simulink model "freego_jump"  (R2022b)
settings: Solver=ode15s  StartTime=0.0  StopTime=20  FixedStep=0.0001  MaxStep=0.04  MinStep=1e-10  RelTol=1e-3  EnableMultiTasking=on
model workspace (MATLAB code in the model file):
  | model = quadruped_robot();
undefined symbols (not defined in the file or in its folder): abad_InitAngle, Fpt, freego, gcontact, gcPosVel, hip_InitAngle, knee_InitAngle, quadruped_robot
libraries: simulink x5, slpidlib x2
(part 1 of 2)
settings Model: Creator=roy  LastModifiedBy=crown133
settings SolverCC: AlgebraicLoopSolver=TrustRegion
settings DataIOCC: SaveFormat=Array  SignalLoggingSaveFormat=ModelDataLogs  ReturnWorkspaceOutputs=off
settings OptimizationCC: ExpressionDepthLimit=2147483647  InitFltsAndDblsToZero=on  LifeSpan=inf
settings DebuggingCC: UnderspecifiedInitializationDetection=Classic  MergeDetectMultiDrivingBlocksExec=none  SolverPrmCheckMsg=warning  FcnCallInpInsideContextMsg=warning  UnconnectedInputMsg=warning  UnconnectedOutputMsg=warning  UnconnectedLineMsg=warning  StateNameClashWarn=warning  SFUnexpectedBacktrackingDiag=warning  SFNoUnconditionalDefaultTransitionDiag=warning  SFExecutionAtInitializationDiag=none  SFMachineParentedDataDiag=warning  ArithmeticOperatorsInVariantConditions=warning
settings HardwareCC: ProdBitPerPointer=32  ProdBitPerSizeT=32  ProdBitPerPtrDiffT=32  ProdLargestAtomicFloat=None  ProdIntDivRoundTo=Undefined  ProdEndianess=Unspecified  ProdWordSize=32  ProdHWDeviceType=32-bit Generic
settings ModelReferenceCC: EnableRefExpFcnMdlSchedulingChecks=on  PropagateSignalLabelsOutOfModel=off
settings SFSimCC: SimUseLocalCustomCode=off  CustomCodeUndefinedFunction=UseInterfaceOnly
settings RTWCC: RTWUseLocalCustomCode=off
settings CodeAppCC: StateflowObjectComments=on
settings GRTTargetCC: TargetLangStandard=C89/C90 (ANSI)  CombineOutputUpdateFcns=off  GRTInterface=on
settings ConfigComp: CovMetricSettings=dw  CovSaveCumulativeToWorkspaceVar=on  CovSaveSingleToWorkspaceVar=on  CovExternalEMLEnable=off

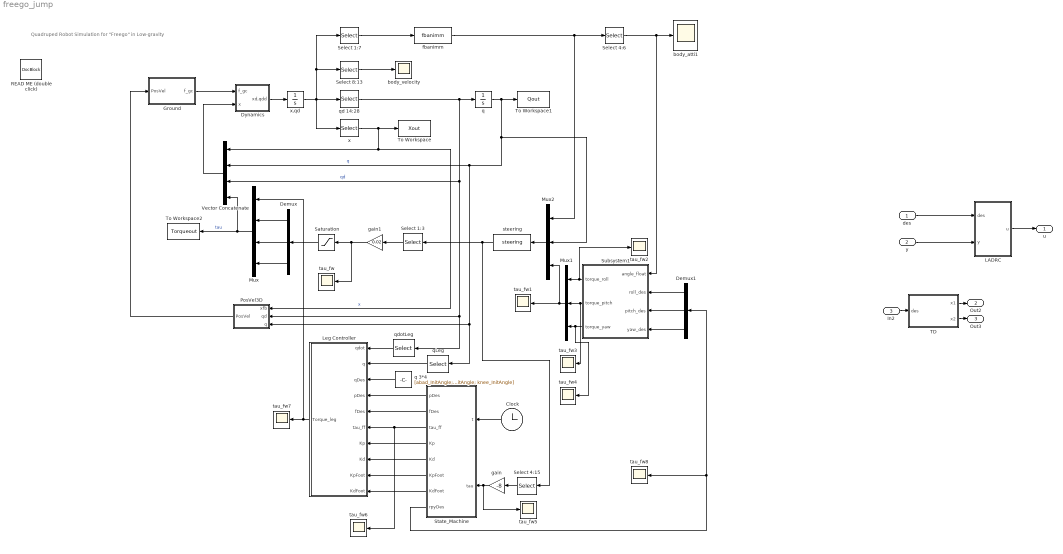
== system freego_jump ==
  note: Quadruped Robot Simulation for "Freego" in Low-gravity
  des : Inport
  y : Inport  Port=2
  In2 : Inport  Port=3
  Clock : Clock
  Demux : Demux  Outputs=3
  Demux1 : Demux  Outputs=3
  Dynamics : Subsystem
  Ground : Subsystem
  LADRC : Subsystem
  Leg Controller : Subsystem
  Mux : Mux
  Mux1 : Mux  Inputs=3
  Mux2 : Mux  Inputs=3
  PosVel3D : Subsystem
  READ ME (double click) : simulink/Model-Wide Utilities/DocBlock  DocumentType=Text
      content=|
      | This Simulink model shows how to use the ground-contact model, which
      | allows you to simulate the effect of physical contact between a rigid-body
      | system and a compliant ground plane.
      |
      | showmotion(quadruped_robot(), tout, fbanim(Xout, Qout))
      |
      | fbanim() 专为showmotion() 设计
  Saturation : Saturate  UpperLimit=1  LowerLimit=-1
  Select 1:3 : Selector  InputPortWidth=15  IndexOptions=Index vector (dialog)  Indices=[1:3]  OutputSizes=1
  Select 1:7 : Selector  InputPortWidth=13+15  IndexOptions=Index vector (dialog)  Indices=[1:7]  OutputSizes=1
  Select 4:15 : Selector  InputPortWidth=15  IndexOptions=Index vector (dialog)  Indices=[4:15]  OutputSizes=1
  Select 4:6 : Selector  InputPortWidth=6  IndexOptions=Index vector (dialog)  Indices=[4:6]  OutputSizes=1
  Select 8:13 : Selector  InputPortWidth=13+15  IndexOptions=Index vector (dialog)  Indices=[8 9 10 11 12 13]  OutputSizes=1
  State_Machine : Subsystem
  Subsystem1 : Subsystem
  TD : Subsystem
  To Workspace : ToWorkspace  VariableName=Xout  SampleTime=-1
  To Workspace1 : ToWorkspace  VariableName=Qout  SampleTime=-1
  To Workspace2 : ToWorkspace  VariableName=Torqueout  SampleTime=-1
  Vector Concatenate : Concatenate  NumInputs=4
  body_atti1 : Scope
  body_velocity : Scope
  fbanimm : MATLABFcn  MATLABFcn=fbanimm  OutputDimensions=6
  gain : Gain  Gain=-8
  gain1 : Gain  Gain=0.02
  q : Integrator  InitialCondition=[freego.q_init]'
  q 3*4 : Constant  Value=[abad_InitAngle; hip_InitAngle; knee_InitAngle]
  qLeg : Selector  InputPortWidth=15  IndexOptions=Index vector (dialog)  Indices=[1:12]  OutputSizes=1
  qd 14:28 : Selector  InputPortWidth=13+15  IndexOptions=Index vector (dialog)  Indices=[14:13+15]  OutputSizes=1
  qdotLeg : Selector  InputPortWidth=15  IndexOptions=Index vector (dialog)  Indices=[1:12]  OutputSizes=1
  steering : MATLABFcn  MATLABFcn=steering  OutputDimensions=15  Output1D=off
  tau_fw{,1..8} (9 alike) : Scope
  x : Selector  InputPortWidth=13+15  IndexOptions=Index vector (dialog)  Indices=[1:13]  OutputSizes=1
  x,qd : Integrator  InitialCondition=[freego.QuatBody, freego.COMLocation, zeros(1,6), zeros(1,15)]'
  u : Outport
  Out2 : Outport  Port=2
  Out3 : Outport  Port=3
  wires:
  PosVel3D/1(PosVel) -> Ground/1(PosVel)
  Dynamics/1(xd,qdd) -> x,qd/1
  Select 8:13/1 -> body_velocity/1
  qd 14:28/1 -> q/1, qdotLeg/1, PosVel3D/2(qd), Vector Concatenate/3  "qd"
  q/1 -> To Workspace1/1, Mux2/2, Vector Concatenate/2, qLeg/1, PosVel3D/3(q)  "q"
  x/1 -> To Workspace/1, Vector Concatenate/1, PosVel3D/1(xfb)  "x"
  Vector Concatenate/1 -> Dynamics/2(x)
  Ground/1(f_gc) -> Dynamics/1(f_gc)
  Mux/1 -> Vector Concatenate/4, To Workspace2/1  "tau"
  des/1 -> LADRC/1(des)
  y/1 -> LADRC/2(y)
  LADRC/1(u) -> u/1
  In2/1 -> TD/1(des)
  TD/2(x2) -> Out3/1
  TD/1(x1) -> Out2/1
  Demux/1 -> Mux/2
  q 3*4/1 -> Leg Controller/3(qDes)
  Leg Controller/1(Torque_leg) -> Mux/1, tau_fw7/1
  qLeg/1 -> Leg Controller/2(q)
  qdotLeg/1 -> Leg Controller/1(qdot)
  Select 1:7/1 -> fbanimm/1
  fbanimm/1 -> Select 4:6/1, Mux2/1
  Select 4:6/1 -> body_atti1/1, Subsystem1/1(angle_float)
  Demux1/2 -> Subsystem1/3(pitch_des)
  Subsystem1/1(torque_roll) -> Mux1/1, tau_fw2/1
  Subsystem1/2(torque_pitch) -> Mux1/2, tau_fw3/1
  Subsystem1/3(torque_yaw) -> Mux1/3, tau_fw4/1
  Mux2/1 -> steering/1
  Mux1/1 -> tau_fw1/1, Mux2/3
  steering/1 -> Select 4:15/1, Select 1:3/1
  Select 1:3/1 -> gain1/1
  gain1/1 -> tau_fw/1, Saturation/1
  Select 4:15/1 -> gain/1
  Demux1/1 -> Subsystem1/2(roll_des)
  Demux1/3 -> Subsystem1/4(yaw_des)
  Saturation/1 -> Demux/1
  Clock/1 -> State_Machine/1(t)
  gain/1 -> tau_fw5/1, State_Machine/2(tau)
  State_Machine/7(KdFoot) -> Leg Controller/10(KdFoot)
  State_Machine/6(KpFoot) -> Leg Controller/9(KpFoot)
  State_Machine/5(Kd) -> Leg Controller/8(Kd)
  State_Machine/4(Kp) -> Leg Controller/7(Kp)
  State_Machine/3(tau_ff) -> tau_fw6/1, Leg Controller/6(tau_ff)
  State_Machine/2(fDes) -> Leg Controller/5(fDes)
  State_Machine/1(pDes) -> Leg Controller/4(pDes)
  State_Machine/8(rpyDes) -> tau_fw8/1, Demux1/1
  Demux/3 -> Mux/4
  Demux/2 -> Mux/3
  x,qd/1 -> x/1, qd 14:28/1, Select 1:7/1, Select 8:13/1

== system freego_jump/Dynamics ==
  f_gc : Inport
  x : Inport  Port=2
  Quadruped_robot Dynamics : MATLABFcn  MATLABFcn=gcFD( quadruped_robot, @FDfb, u )  OutputDimensions=[13+15 1]  OutputSignalType=real  Output1D=off
  Reshape : Reshape  OutputDimensionality=Column vector (2-D)
  Vector Concatenate : Concatenate
  xd,qdd : Outport
  wires:
  Vector Concatenate/1 -> Quadruped_robot Dynamics/1
  Quadruped_robot Dynamics/1 -> xd,qdd/1
  f_gc/1 -> Reshape/1
  x/1 -> Vector Concatenate/1
  Reshape/1 -> Vector Concatenate/2

== system freego_jump/Ground ==
  PosVel : Inport
  3D Ground Contact : Subsystem  mask(3D Nonlinear Ground Contact with Friction){K=1e6, D=2000, mu=0.35, np=16}
      mask prompts: K "Stiffness (K)"; D "Damping (D)"; mu "Coefficient of Friction (mu)"; np "Number of Contact Points"
      mask help:
      | Given two 3xnp arrays containing contact-point positions and
      | velocities, calculate the 3xnp array of ground-reaction forces
      | acting on those points. Also calculate 1xnp boolean vectors
      | in_ctact (true if normal force >0) and sticking (true if inside
      | or on boundary of friction cone).  Zero-crossing detection is
      | enabled at both make/break contact and stick/slip transitions.
  READ ME : simulink/Model-Wide Utilities/DocBlock  DocumentType=Text
      content=|
      | This subsystem implements the Simulink ground-contact model in 3D.  The
      | input is a 6x(npt) matrix such that column i contains the 3D position (top
      | 3 elements) and linear velocity (bottom 3 elements) of ground-contact
      | point number i (i.e., the i^th point defined in the "gc" field of the
      | system model data structure).  The output is a 6x(npt) matrix such that
      | column i is the spatial force acting on point number i.  All quantities
      | are expressed in base (body 0) coordinates.
      |
      | The first thing that happens is that the input matrix is split into
      | separate position and velocity matrices.  Both are then sent to the "3D
      | Ground Contact" subsystem, which calculates the force acting on each
      | point.  The "force" output is a 3x(npt) matrix of linear forces, which is
      | converted to a matrix of spatial forces by the final block in the
      | subsystem.  The other two outputs are 1x(npt) arrays of Boolean variables
      | such that in_ctact(i) is true if point i is in contact with the ground
      | (meaning that it is experiencing a nonzero force) and sticking(i) is true
      | if point i is sticking (due to friction) to the ground.
      |
      | The subsystem "3D Ground Contact" is a masked subsystem.  If you
      | double-click on this block then you will get a dialog window displaying
      | the following parameters: Stiffness (K), Damping (D), coefficient of
      | friction (mu), and Number of Contact Points.  The first three must be
      | strictly-positive scalars, and the fourth must equal the number of points
      | defined in the "gc" field of the system model data structure.  The current
      | settings of K, D and mu correspond to a soft, very slippery plastic
      | surface.  Increasing K will make it harder, and increasing the ratio K/D
      | will make it bouncier, but be aware that both increase the stiffness of
      | the differential equations that Simulink is solving, meaning that Simulink
      | will be forced to take smaller steps.  A typical value of mu for a safe
      | (non-slip) floor is 0.5.
      |
      | To see how this subsystem is implemented, you will have to look under the
      | mask.  You can do that by right-clicking on the block and selecting the
      | menu option "Look Under Mask".  There, you will find that this block is
      | based on the function gcontact, and you will also find a bit more
      | documentation.
  Terminator : Terminator
  Terminator1 : Terminator
  convert 3D to spatial forces : Subsystem
  select pos : Selector  NumberOfDimensions=2  InputPortWidth=3  IndexOptions=Index vector (dialog),Select all  Indices=[1 2 3],1  OutputSizes=1,1
  select vel : Selector  NumberOfDimensions=2  InputPortWidth=3  IndexOptions=Index vector (dialog),Select all  Indices=[4 5 6],1  OutputSizes=1,1
  f_gc : Outport
  wires:
  PosVel/1 -> select pos/1, select vel/1
  select pos/1 -> convert 3D to spatial forces/1(pos), 3D Ground Contact/1(pos)
  convert 3D to spatial forces/1(force6D) -> f_gc/1
  select vel/1 -> 3D Ground Contact/2(vel)
  3D Ground Contact/1(force) -> convert 3D to spatial forces/2(force3D)
  3D Ground Contact/2(in_ctact) -> Terminator/1
  3D Ground Contact/3(sticking) -> Terminator1/1

== system freego_jump/LADRC ==
  des : Inport
  y : Inport  Port=2
  1/b0 : Gain
  LESO3 : Subsystem
  PID Controller : slpidlib/PID Controller  Controller=PID  Form=Parallel  TimeDomain=Continuous-time  UseExternalTs=off  SampleTime=-1  IntegratorMethod=Forward Euler  FilterMethod=Forward Euler  ControllerParametersSource=internal  P=10  I=0.01  UseKiTs=off  D=1  N=100  UseFilter=on  TunerSelectOption=Transfer Function Based (PID Tuner App)  InitialConditionSource=internal  InitialConditionForIntegrator=0  InitialConditionForFilter=0  DifferentiatorICPrevScaledInput=0  ExternalReset=none  TrackingMode=off  Kt=1  LimitOutput=off  SatLimitsSource=internal  UpperSaturationLimit=inf  LowerSaturationLimit=-inf  LinearizeAsGain=on  AntiWindupMode=none  Kb=1  LimitIntegrator=off  UpperIntegratorSaturationLimit=inf  LowerIntegratorSaturationLimit=-inf  POutMin=[]  POutMax=[]  IOutMin=[]  IOutMax=[]  DOutMin=[]  DOutMax=[]  NOutMin=[]  NOutMax=[]  SumOutMin=[]  SumOutMax=[]  SaturationOutMin=[]  SaturationOutMax=[]  PParamMin=[]  PParamMax=[]  IParamMin=[]  IParamMax=[]  DParamMin=[]  DParamMax=[]  NParamMin=[]  NParamMax=[]  KbParamMin=[]  KbParamMax=[]  KtParamMin=[]  KtParamMax=[]  KbOutMin=[]  KbOutMax=[]  KtOutMin=[]  KtOutMax=[]  IntegratorOutMin=[]  IntegratorOutMax=[]  FilterOutMin=[]  FilterOutMax=[]  SumI1OutMin=[]  SumI1OutMax=[]  SumI2OutMin=[]  SumI2OutMax=[]  SumI3OutMin=[]  SumI3OutMax=[]  SumI4OutMin=[]  SumI4OutMax=[]  SumDOutMin=[]  SumDOutMax=[]  DifferentiatorOutMin=[]  DifferentiatorOutMax=[]  FilterDiffOutCoefMin=[]  FilterDiffOutCoefMax=[]  ReciprocalOutMin=[]  ReciprocalOutMax=[]  SumDenOutMin=[]  SumDenOutMax=[]  SumNumOutMin=[]  SumNumOutMax=[]  DivideOutMin=[]  DivideOutMax=[]  UdiffTsProdOutMin=[]  UdiffTsProdOutMax=[]  NTsProdOutMin=[]  NTsProdOutMax=[]  UintegralTsProdOutMin=[]  UintegralTsProdOutMax=[]  UngainTsProdOutMin=[]  UngainTsProdOutMax=[]  ClampingZeroOutDataTypeStr=Inherit: Inherit via back propagation  ClampingZeroOutMin=[]  ClampingZeroOutMax=[]  FilterDenConstantOutDataTypeStr=Inherit: Inherit via back propagation  FilterDenConstantOutMin=[]  FilterDenConstantOutMax=[]  PCopyOutDataTypeStr=Inherit: Inherit via back propagation  PCopyOutMin=[]  PCopyOutMax=[]  NCopyOutDataTypeStr=Inherit: Inherit via back propagation  NCopyOutMin=[]  NCopyOutMax=[]  IntegratorContinuousStateAttributes=''  IntegratorStateMustResolveToSignalObject=off  IntegratorRTWStateStorageClass=Auto  FilterContinuousStateAttributes=''  FilterStateMustResolveToSignalObject=off  FilterRTWStateStorageClass=Auto  ParallelPVariant=InternalParameters  IdealPVariant=Disabled  IVariant=InternalParameters  DVariant=InternalParameters  IntegratorVariant=Continuous  SatVariant=Disabled  AWVariant=Passthrough  PCopyVariant=Disabled  TRVariant=Disabled  FdbkBlocksVariant=Forward  IdealPFdbkVariant=Disabled  SatFdbkVariant=Disabled  DerivativeFilterVariant=ContFilter  NVariant=InternalParameters  NCopyVariant=Disabled  FilterICVariant=InternalICsFilter  IntegratorICVariant=InternalICs  ExternalResetVariant=Disabled  TRSumVariant=Passthrough  SumFdbkVariant=Disabled  SumVariant=Sum_PID  TsampFilterVariant=InternalTs  TsampNgainVariant=Passthrough  TsampIntegralVariant=Passthrough  ExternalSaturationOutDataTypeStr=Inherit: Same as second input
  PID Controller1 : slpidlib/PID Controller  Controller=PID  Form=Parallel  TimeDomain=Continuous-time  UseExternalTs=off  SampleTime=-1  IntegratorMethod=Forward Euler  FilterMethod=Forward Euler  ControllerParametersSource=internal  P=10  I=0.01  UseKiTs=off  D=1  N=100  UseFilter=on  TunerSelectOption=Transfer Function Based (PID Tuner App)  InitialConditionSource=internal  InitialConditionForIntegrator=0  InitialConditionForFilter=0  DifferentiatorICPrevScaledInput=0  ExternalReset=none  TrackingMode=off  Kt=1  LimitOutput=off  SatLimitsSource=internal  UpperSaturationLimit=inf  LowerSaturationLimit=-inf  LinearizeAsGain=on  AntiWindupMode=none  Kb=1  LimitIntegrator=off  UpperIntegratorSaturationLimit=inf  LowerIntegratorSaturationLimit=-inf  POutMin=[]  POutMax=[]  IOutMin=[]  IOutMax=[]  DOutMin=[]  DOutMax=[]  NOutMin=[]  NOutMax=[]  SumOutMin=[]  SumOutMax=[]  SaturationOutMin=[]  SaturationOutMax=[]  PParamMin=[]  PParamMax=[]  IParamMin=[]  IParamMax=[]  DParamMin=[]  DParamMax=[]  NParamMin=[]  NParamMax=[]  KbParamMin=[]  KbParamMax=[]  KtParamMin=[]  KtParamMax=[]  KbOutMin=[]  KbOutMax=[]  KtOutMin=[]  KtOutMax=[]  IntegratorOutMin=[]  IntegratorOutMax=[]  FilterOutMin=[]  FilterOutMax=[]  SumI1OutMin=[]  SumI1OutMax=[]  SumI2OutMin=[]  SumI2OutMax=[]  SumI3OutMin=[]  SumI3OutMax=[]  SumI4OutMin=[]  SumI4OutMax=[]  SumDOutMin=[]  SumDOutMax=[]  DifferentiatorOutMin=[]  DifferentiatorOutMax=[]  FilterDiffOutCoefMin=[]  FilterDiffOutCoefMax=[]  ReciprocalOutMin=[]  ReciprocalOutMax=[]  SumDenOutMin=[]  SumDenOutMax=[]  SumNumOutMin=[]  SumNumOutMax=[]  DivideOutMin=[]  DivideOutMax=[]  UdiffTsProdOutMin=[]  UdiffTsProdOutMax=[]  NTsProdOutMin=[]  NTsProdOutMax=[]  UintegralTsProdOutMin=[]  UintegralTsProdOutMax=[]  UngainTsProdOutMin=[]  UngainTsProdOutMax=[]  ClampingZeroOutDataTypeStr=Inherit: Inherit via back propagation  ClampingZeroOutMin=[]  ClampingZeroOutMax=[]  FilterDenConstantOutDataTypeStr=Inherit: Inherit via back propagation  FilterDenConstantOutMin=[]  FilterDenConstantOutMax=[]  PCopyOutDataTypeStr=Inherit: Inherit via back propagation  PCopyOutMin=[]  PCopyOutMax=[]  NCopyOutDataTypeStr=Inherit: Inherit via back propagation  NCopyOutMin=[]  NCopyOutMax=[]  IntegratorContinuousStateAttributes=''  IntegratorStateMustResolveToSignalObject=off  IntegratorRTWStateStorageClass=Auto  FilterContinuousStateAttributes=''  FilterStateMustResolveToSignalObject=off  FilterRTWStateStorageClass=Auto  ParallelPVariant=InternalParameters  IdealPVariant=Disabled  IVariant=InternalParameters  DVariant=InternalParameters  IntegratorVariant=Continuous  SatVariant=Disabled  AWVariant=Passthrough  PCopyVariant=Disabled  TRVariant=Disabled  FdbkBlocksVariant=Forward  IdealPFdbkVariant=Disabled  SatFdbkVariant=Disabled  DerivativeFilterVariant=ContFilter  NVariant=InternalParameters  NCopyVariant=Disabled  FilterICVariant=InternalICsFilter  IntegratorICVariant=InternalICs  ExternalResetVariant=Disabled  TRSumVariant=Passthrough  SumFdbkVariant=Disabled  SumVariant=Sum_PID  TsampFilterVariant=InternalTs  TsampNgainVariant=Passthrough  TsampIntegralVariant=Passthrough  ExternalSaturationOutDataTypeStr=Inherit: Same as second input
  Sum1 : Sum  Inputs=|+-
  Sum2 : Sum  Inputs=|+-
  Sum3 : Sum  Inputs=+|+
  Sum4 : Sum  Inputs=|+-
  "TD3 " : Subsystem
  b0 : Gain
  u : Outport
  wires:
  des/1 -> "TD3 "/1(des)
  Sum3/1 -> Sum4/1
  1/b0/1 -> Sum4/2
  PID Controller1/1 -> Sum3/2
  y/1 -> LESO3/1(y)
  Sum2/1 -> PID Controller1/1
  LESO3/3(z3) -> 1/b0/1
  PID Controller/1 -> Sum3/1
  "TD3 "/2(x2) -> Sum2/1
  LESO3/2(z2) -> Sum2/2
  "TD3 "/1(x1) -> Sum1/1
  Sum1/1 -> PID Controller/1
  b0/1 -> LESO3/2(b0u)
  LESO3/1(z1) -> Sum1/2
  Sum4/1 -> u/1, b0/1

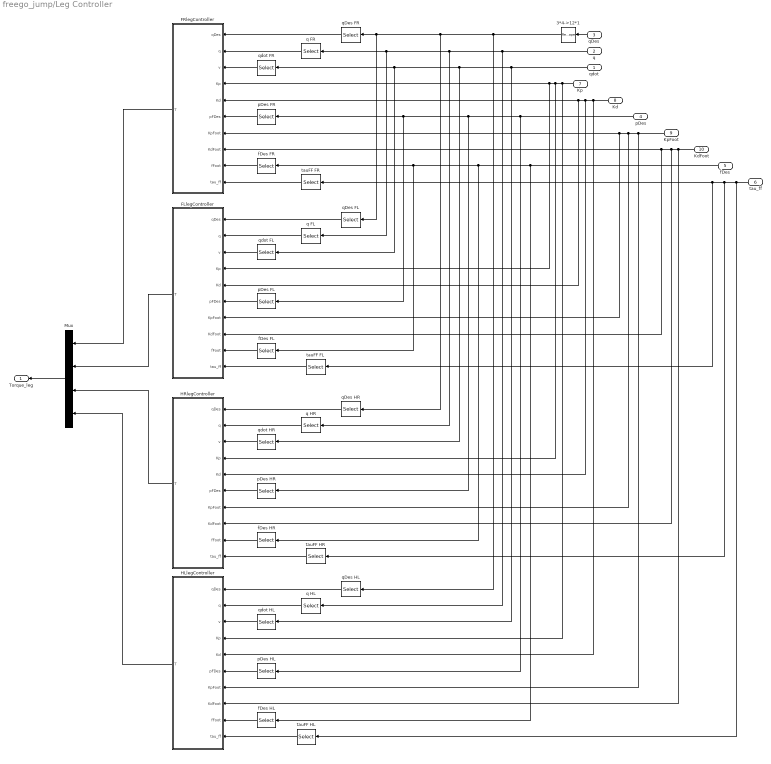
== system freego_jump/Leg Controller ==
  qdot : Inport
  q : Inport  Port=2
  qDes : Inport  Port=3
  pDes : Inport  Port=4
  fDes : Inport  Port=5
  tau_ff : Inport  Port=6
  Kp : Inport  Port=7
  Kd : Inport  Port=8
  KpFoot : Inport  Port=9
  KdFoot : Inport  Port=10
  3*4->12*1 : Reshape  OutputDimensionality=Column vector (2-D)
  FLlegController : Subsystem
  FRlegController : Subsystem
  HLlegController : Subsystem
  HRlegController : Subsystem
  Mux : Mux
  fDes FL : Selector  InputPortWidth=12  IndexOptions=Index vector (dialog)  Indices=[4:6]  OutputSizes=1
  fDes FR : Selector  InputPortWidth=12  IndexOptions=Index vector (dialog)  Indices=[1:3]  OutputSizes=1
  fDes HL : Selector  InputPortWidth=12  IndexOptions=Index vector (dialog)  Indices=[10:12]  OutputSizes=1
  fDes HR : Selector  InputPortWidth=12  IndexOptions=Index vector (dialog)  Indices=[7:9]  OutputSizes=1
  pDes FL : Selector  InputPortWidth=12  IndexOptions=Index vector (dialog)  Indices=[4:6]  OutputSizes=1
  pDes FR : Selector  InputPortWidth=12  IndexOptions=Index vector (dialog)  Indices=[1:3]  OutputSizes=1
  pDes HL : Selector  InputPortWidth=12  IndexOptions=Index vector (dialog)  Indices=[10:12]  OutputSizes=1
  pDes HR : Selector  InputPortWidth=12  IndexOptions=Index vector (dialog)  Indices=[7:9]  OutputSizes=1
  q FL : Selector  InputPortWidth=12  IndexOptions=Index vector (dialog)  Indices=[4:6]  OutputSizes=1
  q FR : Selector  InputPortWidth=12  IndexOptions=Index vector (dialog)  Indices=[1:3]  OutputSizes=1
  q HL : Selector  InputPortWidth=12  IndexOptions=Index vector (dialog)  Indices=[10:12]  OutputSizes=1
  q HR : Selector  InputPortWidth=12  IndexOptions=Index vector (dialog)  Indices=[7:9]  OutputSizes=1
  qDes FL : Selector  InputPortWidth=12  IndexOptions=Index vector (dialog)  Indices=[4:6]  OutputSizes=1
  qDes FR : Selector  InputPortWidth=12  IndexOptions=Index vector (dialog)  Indices=[1:3]  OutputSizes=1
  qDes HL : Selector  InputPortWidth=12  IndexOptions=Index vector (dialog)  Indices=[10:12]  OutputSizes=1
  qDes HR : Selector  InputPortWidth=12  IndexOptions=Index vector (dialog)  Indices=[7:9]  OutputSizes=1
  qdot FL : Selector  InputPortWidth=12  IndexOptions=Index vector (dialog)  Indices=[4:6]  OutputSizes=1
  qdot FR : Selector  InputPortWidth=12  IndexOptions=Index vector (dialog)  Indices=[1:3]  OutputSizes=1
  qdot HL : Selector  InputPortWidth=12  IndexOptions=Index vector (dialog)  Indices=[10:12]  OutputSizes=1
  qdot HR : Selector  InputPortWidth=12  IndexOptions=Index vector (dialog)  Indices=[7:9]  OutputSizes=1
  tauFF FL : Selector  InputPortWidth=12  IndexOptions=Index vector (dialog)  Indices=[4:6]  OutputSizes=1
  tauFF FR : Selector  InputPortWidth=12  IndexOptions=Index vector (dialog)  Indices=[1:3]  OutputSizes=1
  tauFF HL : Selector  InputPortWidth=12  IndexOptions=Index vector (dialog)  Indices=[10:12]  OutputSizes=1
  tauFF HR : Selector  InputPortWidth=12  IndexOptions=Index vector (dialog)  Indices=[7:9]  OutputSizes=1
  Torque_leg : Outport
  wires:
  q FR/1 -> FRlegController/2(q)
  qDes/1 -> 3*4->12*1/1
  qdot/1 -> qdot FL/1, qdot FR/1, qdot HR/1, qdot HL/1
  qdot FR/1 -> FRlegController/3(v)
  q FL/1 -> FLlegController/2(q)
  Kd/1 -> HLlegController/5(Kd), HRlegController/5(Kd), FRlegController/5(Kd), FLlegController/5(Kd)
  KpFoot/1 -> FRlegController/7(KpFoot), FLlegController/7(KpFoot), HRlegController/7(KpFoot), HLlegController/7(KpFoot)
  qDes FL/1 -> FLlegController/1(qDes)
  pDes FL/1 -> FLlegController/6(pFDes)
  q/1 -> q FL/1, q FR/1, q HR/1, q HL/1
  qdot FL/1 -> FLlegController/3(v)
  qDes FR/1 -> FRlegController/1(qDes)
  pDes FR/1 -> FRlegController/6(pFDes)
  3*4->12*1/1 -> qDes FL/1, qDes FR/1, qDes HR/1, qDes HL/1
  pDes/1 -> pDes FL/1, pDes FR/1, pDes HR/1, pDes HL/1
  q HR/1 -> HRlegController/2(q)
  qDes HR/1 -> HRlegController/1(qDes)
  pDes HR/1 -> HRlegController/6(pFDes)
  qdot HR/1 -> HRlegController/3(v)
  q HL/1 -> HLlegController/2(q)
  Kp/1 -> HLlegController/4(Kp), HRlegController/4(Kp), FLlegController/4(Kp), FRlegController/4(Kp)
  KdFoot/1 -> FRlegController/8(KdFoot), FLlegController/8(KdFoot), HRlegController/8(KdFoot), HLlegController/8(KdFoot)
  fDes/1 -> fDes HL/1, fDes HR/1, fDes FL/1, fDes FR/1
  qDes HL/1 -> HLlegController/1(qDes)
  pDes HL/1 -> HLlegController/6(pFDes)
  qdot HL/1 -> HLlegController/3(v)
  Mux/1 -> Torque_leg/1
  FRlegController/1(T) -> Mux/1
  FLlegController/1(T) -> Mux/2
  HRlegController/1(T) -> Mux/3
  HLlegController/1(T) -> Mux/4
  fDes FR/1 -> FRlegController/9(fFoot)
  fDes FL/1 -> FLlegController/9(fFoot)
  fDes HR/1 -> HRlegController/9(fFoot)
  fDes HL/1 -> HLlegController/9(fFoot)
  tauFF FL/1 -> FLlegController/10(tau_ff)
  tauFF HR/1 -> HRlegController/10(tau_ff)
  tauFF HL/1 -> HLlegController/10(tau_ff)
  tauFF FR/1 -> FRlegController/10(tau_ff)
  tau_ff/1 -> tauFF HL/1, tauFF HR/1, tauFF FL/1, tauFF FR/1

== system freego_jump/PosVel3D ==
  note: The constant supplies the
      | argument for rollingdisc
  xfb : Inport
  qd : Inport  Port=2
  q : Inport  Port=3
  Vector Concatenate1 : Concatenate  NumInputs=3
  gcPosVel : MATLABFcn  MATLABFcn=gcPosVel( quadruped_robot(), u(1:13), u(14:28), u(29:43))  OutputDimensions=[6 16]  OutputSignalType=real  Output1D=off
  PosVel : Outport
  wires:
  gcPosVel/1 -> PosVel/1
  Vector Concatenate1/1 -> gcPosVel/1
  q/1 -> Vector Concatenate1/2
  xfb/1 -> Vector Concatenate1/1
  qd/1 -> Vector Concatenate1/3

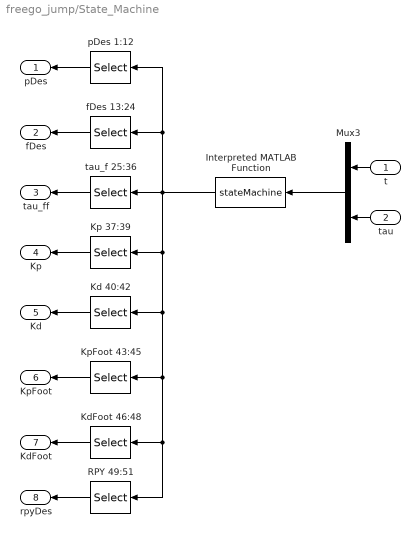
== system freego_jump/State_Machine ==
  t : Inport
  tau : Inport  Port=2
  Interpreted MATLAB Function : MATLABFcn  MATLABFcn=stateMachine  OutputDimensions=51
  Kd 40:42 : Selector  InputPortWidth=51  IndexOptions=Index vector (dialog)  Indices=[40:42]  OutputSizes=1
  KdFoot 46:48 : Selector  InputPortWidth=51  IndexOptions=Index vector (dialog)  Indices=[46:48]  OutputSizes=1
  Kp 37:39 : Selector  InputPortWidth=51  IndexOptions=Index vector (dialog)  Indices=[37:39]  OutputSizes=1
  KpFoot 43:45 : Selector  InputPortWidth=51  IndexOptions=Index vector (dialog)  Indices=[43:45]  OutputSizes=1
  Mux3 : Mux  Inputs=2
  RPY 49:51 : Selector  InputPortWidth=51  IndexOptions=Index vector (dialog)  Indices=[49:51]  OutputSizes=1
  fDes 13:24 : Selector  InputPortWidth=51  IndexOptions=Index vector (dialog)  Indices=[13:24]  OutputSizes=1
  pDes 1:12 : Selector  InputPortWidth=51  IndexOptions=Index vector (dialog)  Indices=[1:12]  OutputSizes=1
  tau_f 25:36 : Selector  InputPortWidth=51  IndexOptions=Index vector (dialog)  Indices=[25:36]  OutputSizes=1
  pDes : Outport
  fDes : Outport  Port=2
  tau_ff : Outport  Port=3
  Kp : Outport  Port=4
  Kd : Outport  Port=5
  KpFoot : Outport  Port=6
  KdFoot : Outport  Port=7
  rpyDes : Outport  Port=8
  wires:
  pDes 1:12/1 -> pDes/1
  fDes 13:24/1 -> fDes/1
  tau/1 -> Mux3/2
  t/1 -> Mux3/1
  tau_f 25:36/1 -> tau_ff/1
  Interpreted MATLAB Function/1 -> pDes 1:12/1, fDes 13:24/1, tau_f 25:36/1, Kp 37:39/1, Kd 40:42/1, KpFoot 43:45/1, RPY 49:51/1, KdFoot 46:48/1
  Mux3/1 -> Interpreted MATLAB Function/1
  Kp 37:39/1 -> Kp/1
  Kd 40:42/1 -> Kd/1
  KpFoot 43:45/1 -> KpFoot/1
  KdFoot 46:48/1 -> KdFoot/1
  RPY 49:51/1 -> rpyDes/1

== system freego_jump/Subsystem1 ==
  angle_float : Inport
  roll_des : Inport  Port=2
  pitch_des : Inport  Port=3
  yaw_des : Inport  Port=4
  Demux : Demux  Outputs=3
  LADRC_Pitch : Subsystem
  LADRC_Roll : Subsystem
  LADRC_Yaw : Subsystem
  p : Gain  Gain=-1
  p1 : Gain  Gain=-1
  p2 : Gain  Gain=-1
  torque_roll : Outport
  torque_pitch : Outport  Port=2
  torque_yaw : Outport  Port=3
  wires:
  LADRC_Yaw/1(u) -> p2/1
  yaw_des/1 -> LADRC_Yaw/1(des)
  pitch_des/1 -> LADRC_Pitch/1(des)
  LADRC_Pitch/1(u) -> p1/1
  angle_float/1 -> Demux/1
  p/1 -> torque_roll/1
  roll_des/1 -> LADRC_Roll/1(des)
  LADRC_Roll/1(u) -> p/1
  Demux/2 -> LADRC_Pitch/2(y)
  Demux/1 -> LADRC_Roll/2(y)
  Demux/3 -> LADRC_Yaw/2(y)
  p1/1 -> torque_pitch/1
  p2/1 -> torque_yaw/1

== system freego_jump/TD ==
  des : Inport
  MATLAB Function1 : MATLAB Function  TreatAsAtomicUnit=on
  Product : Product
  Product1 : Product
  Sum : Sum  Inputs=+-|
  h : Constant
  r : Constant  Value=10000000000000000000000000
  sx1 : Integrator
  sx2 : Integrator
  x1 : Outport
  x2 : Outport  Port=2
  wires:
  sx2/1 -> MATLAB Function1/2(x2), x2/1, Product1/1
  h/1 -> MATLAB Function1/4(h), Product/2, Product1/2  "h"
  Product/1 -> sx2/1
  MATLAB Function1/1(fh) -> Product/1
  sx1/1 -> Sum/1, x1/1
  r/1 -> MATLAB Function1/3(r)
  Product1/1 -> sx1/1
  Sum/1 -> MATLAB Function1/1(x1)
  des/1 -> Sum/2

== system freego_jump/Ground/3D Ground Contact ==
  pos : Inport
  vel : Inport  Port=2
  Compare To Constant : simulink/Logic and Bit Operations/Compare To Constant  relop=<=  const=1  OutDataTypeStr=boolean
  Compare To Zero : simulink/Logic and Bit Operations/Compare To Zero  relop=>  OutDataTypeStr=boolean
  K,D,mu : Constant  Value=[ [K; D; mu] zeros(3,np-1) ]  VectorParams1D=off
  READ ME : simulink/Model-Wide Utilities/DocBlock  DocumentType=Text
      content=|
      | The constant block supplies the parameters K, D and mu to the function
      | gcontact.  This is necessary because K, D and mu are defined in the
      | workspace of this particular masked subsystem, but the executable
      | expression in the "MATLAB Function" block does not have access to this
      | workspace, so the symbols K, D and mu cannot appear directly in the
      | executable expression.
      |
      | The ">0" block and the "<=1" block both have zero-crossing enabled.  The
      | former detects transitions between contact and non-contact, whereas the
      | latter detects transitions between sticking (due to friction) and
      | slipping.  A point can be sticking only if it is also in contact.  A
      | zero-crossing event occurs whenever any one point makes a transition.
      |
      | The state variable, u, is a 2x(np) matrix containing the horizontal
      | component of the local ground deformation for each point.  This quantity
      | is used to calculate the tangential (i.e., frictional) component of the
      | ground reaction force.
      |
      | When a point loses contact, its associated state variable, u(:,i), decays
      | to zero with a time constant of D/K.  If this ratio is small then the
      | corresponding differential equation is fast, and it is necessary to use
      | small integration time steps.  For example, if K=1e6 and D=2000 then
      | D/K=0.002 and u(:,i) decays in proportion to exp(-500t).  Increasing K
      | makes the surface stiffer, and decreasing D/K makes it bouncier, but the
      | latter also makes the post-contact recovery faster.  The degree of
      | bounciness depends on the mass of the impacting body: a heavier body will
      | bounce more.
      |
      | To adapt this subsystem to work in 2D, the only things that change are the
      | row dimensions of various matrices.  You will have to alter the row
      | selections in the executable expression in the "MATLAB Function" block,
      | and also the dimensions of its output matrix, and you will have to change
      | the row selections in the various "select" blocks.
      |
      | For more information, see "The Simulink Ground Contact Model" in the
      | spatial_v2 documentation directory.
  Vector Concatenate : Concatenate  NumInputs=4  Mode=Multidimensional array
  gcontact : MATLABFcn  MATLABFcn=gcontact( u(1,1), u(2,1), u(3,1), u(4:6,:), u(7:9,:), u(10:11,:) )  OutputDimensions=[6 np]  OutputSignalType=real  Output1D=off
  select fcone : Selector  NumberOfDimensions=2  InputPortWidth=3  IndexOptions=Index vector (dialog),Select all  Indices=[6],1  OutputSizes=1,1
  select force : Selector  NumberOfDimensions=2  InputPortWidth=3  IndexOptions=Index vector (dialog),Select all  Indices=[1 2 3],1  OutputSizes=1,1
  select fz : Selector  NumberOfDimensions=2  InputPortWidth=3  IndexOptions=Index vector (dialog),Select all  Indices=[3],1  OutputSizes=1,1
  select ud : Selector  NumberOfDimensions=2  InputPortWidth=3  IndexOptions=Index vector (dialog),Select all  Indices=[4 5],1  OutputSizes=1,1
  u : Integrator
  force : Outport
  in_ctact : Outport  Port=2
  sticking : Outport  Port=3
  wires:
  Vector Concatenate/1 -> gcontact/1
  select ud/1 -> u/1
  gcontact/1 -> select fz/1, select ud/1, select fcone/1, select force/1
  select force/1 -> force/1
  select fz/1 -> Compare To Zero/1
  Compare To Zero/1 -> in_ctact/1
  select fcone/1 -> Compare To Constant/1
  Compare To Constant/1 -> sticking/1
  u/1 -> Vector Concatenate/4
  vel/1 -> Vector Concatenate/3
  pos/1 -> Vector Concatenate/2
  K,D,mu/1 -> Vector Concatenate/1

== system freego_jump/Ground/convert 3D to spatial forces ==
  note: calculate a 6*npt matrix of spatial force vectors (one per column)
      | from a 3*npt matrix of position vectors specifying the points
      | through which the forces act, and a 3*npt matrix of force vectors
  pos : Inport
  force3D : Inport  Port=2
  Fpt : MATLABFcn  MATLABFcn=Fpt( u(4:6,:), u(1:3,:) )  OutputSignalType=real  Output1D=off
  Matrix Concatenate : Concatenate  Mode=Multidimensional array
  force6D : Outport
  wires:
  force3D/1 -> Matrix Concatenate/2
  pos/1 -> Matrix Concatenate/1
  Matrix Concatenate/1 -> Fpt/1
  Fpt/1 -> force6D/1

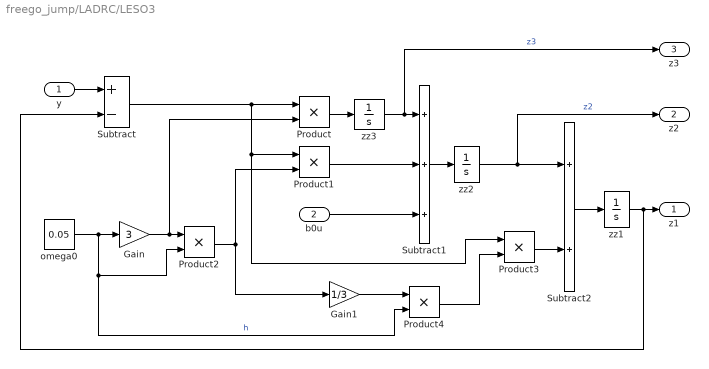
== system freego_jump/LADRC/LESO3 ==
  y : Inport
  b0u : Inport  Port=2
  Gain : Gain  Gain=3
  Gain1 : Gain  Gain=1/3
  Product{,1..4} (5 alike) : Product
  Subtract : Sum  Inputs=+-
  Subtract1 : Sum  Inputs=+++
  Subtract2 : Sum
  omega0 : Constant  Value=0.05
  zz1 : Integrator
  zz2 : Integrator
  zz3 : Integrator
  z1 : Outport
  z2 : Outport  Port=2
  z3 : Outport  Port=3
  wires:
  y/1 -> Subtract/1
  Subtract/1 -> Product/1, Product3/1, Product1/1
  omega0/1 -> Gain/1, Product4/2, Product2/2  "h"
  Gain/1 -> Product/2, Product2/1
  Product/1 -> zz3/1
  zz3/1 -> z3/1, Subtract1/1  "z3"
  b0u/1 -> Subtract1/3
  Product1/1 -> Subtract1/2
  Product2/1 -> Gain1/1, Product1/2
  Subtract1/1 -> zz2/1
  zz2/1 -> Subtract2/1, z2/1  "z2"
  zz1/1 -> Subtract/2, z1/1
  Product3/1 -> Subtract2/2
  Product4/1 -> Product3/2
  Subtract2/1 -> zz1/1
  Gain1/1 -> Product4/1

== system freego_jump/LADRC/TD3  ==
  des : Inport
  Gain : Gain  Gain=-1
  MATLAB Function1 : MATLAB Function  TreatAsAtomicUnit=on
  Product : Product
  d : Constant  Value=0.05
  r : Constant  Value=300
  sx1 : Integrator
  sx2 : Integrator
  x1 : Outport
  x2 : Outport  Port=2
  wires:
  d/1 -> MATLAB Function1/5(d)  "h"
  Product/1 -> sx2/1
  MATLAB Function1/1(f) -> Product/1
  sx1/1 -> MATLAB Function1/1(x1), x1/1
  r/1 -> Gain/1, MATLAB Function1/4(r)
  sx2/1 -> MATLAB Function1/2(x2), sx1/1, x2/1
  des/1 -> MATLAB Function1/3(u)
  Gain/1 -> Product/2

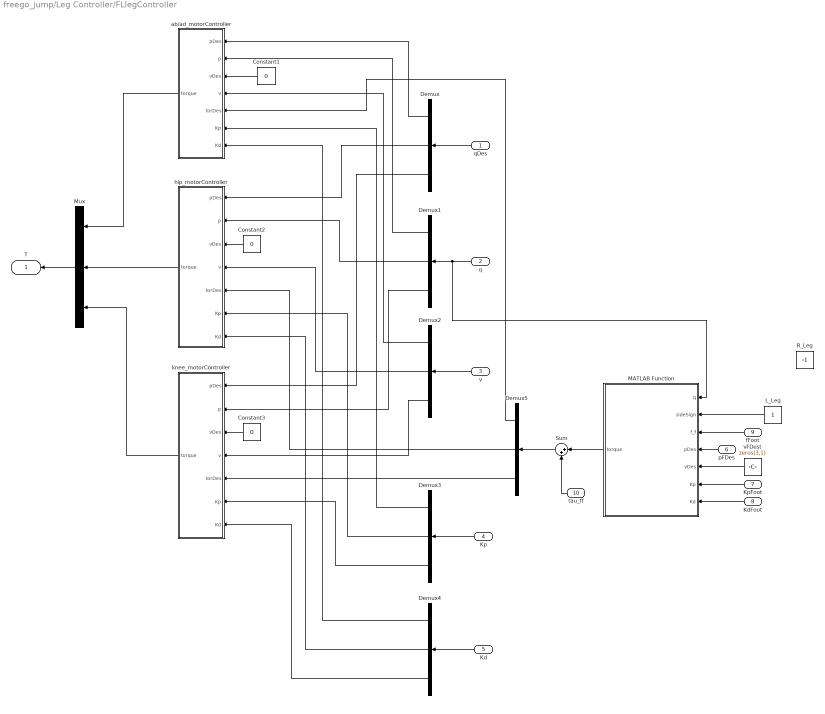
== system freego_jump/Leg Controller/FLlegController ==
  qDes : Inport
  q : Inport  Port=2
  v : Inport  Port=3
  Kp : Inport  Port=4
  Kd : Inport  Port=5
  pFDes : Inport  Port=6
  KpFoot : Inport  Port=7
  KdFoot : Inport  Port=8
  fFoot : Inport  Port=9
  tau_ff : Inport  Port=10
  Constant1 : Constant  Value=0
  Constant2 : Constant  Value=0
  Constant3 : Constant  Value=0
  Demux{,1..5} (6 alike) : Demux  Outputs=3
  L_Leg : Constant
  MATLAB Function : MATLAB Function  TreatAsAtomicUnit=on
  Mux : Mux  Inputs=3
  R_Leg : Constant  Value=-1
  Sum : Sum  Inputs=|++
  ab/ad_motorController : Subsystem
  hip_motorController : Subsystem
  knee_motorController : Subsystem
  vFDest : Constant  Value=zeros(3,1)
  T : Outport
  wires:
  Demux/1 -> ab/ad_motorController/1(pDes)
  Demux1/1 -> ab/ad_motorController/2(p)
  Demux2/1 -> ab/ad_motorController/4(v)
  Demux3/1 -> ab/ad_motorController/6(Kp)
  Demux5/1 -> ab/ad_motorController/5(torDes)
  Constant1/1 -> ab/ad_motorController/3(vDes)
  Demux4/1 -> ab/ad_motorController/7(Kd)
  ab/ad_motorController/1(torque) -> Mux/1
  Constant2/1 -> hip_motorController/3(vDes)
  Demux2/2 -> hip_motorController/4(v)
  Demux/2 -> hip_motorController/1(pDes)
  Demux1/3 -> knee_motorController/2(p)
  Demux5/2 -> hip_motorController/5(torDes)
  Demux3/2 -> hip_motorController/6(Kp)
  Demux5/3 -> knee_motorController/5(torDes)
  Demux/3 -> knee_motorController/1(pDes)
  Constant3/1 -> knee_motorController/3(vDes)
  Demux4/2 -> hip_motorController/7(Kd)
  hip_motorController/1(torque) -> Mux/2
  Demux3/3 -> knee_motorController/6(Kp)
  Demux1/2 -> hip_motorController/2(p)
  knee_motorController/1(torque) -> Mux/3
  Demux4/3 -> knee_motorController/7(Kd)
  qDes/1 -> Demux/1
  q/1 -> MATLAB Function/1(q), Demux1/1
  v/1 -> Demux2/1
  Demux2/3 -> knee_motorController/4(v)
  Kp/1 -> Demux3/1
  Kd/1 -> Demux4/1
  Mux/1 -> T/1
  fFoot/1 -> MATLAB Function/3(f_f)
  KdFoot/1 -> MATLAB Function/7(Kd)
  KpFoot/1 -> MATLAB Function/6(Kp)
  vFDest/1 -> MATLAB Function/5(vDes)
  pFDes/1 -> MATLAB Function/4(pDes)
  L_Leg/1 -> MATLAB Function/2(sideSign)
  tau_ff/1 -> Sum/2
  MATLAB Function/1(torque) -> Sum/1
  Sum/1 -> Demux5/1

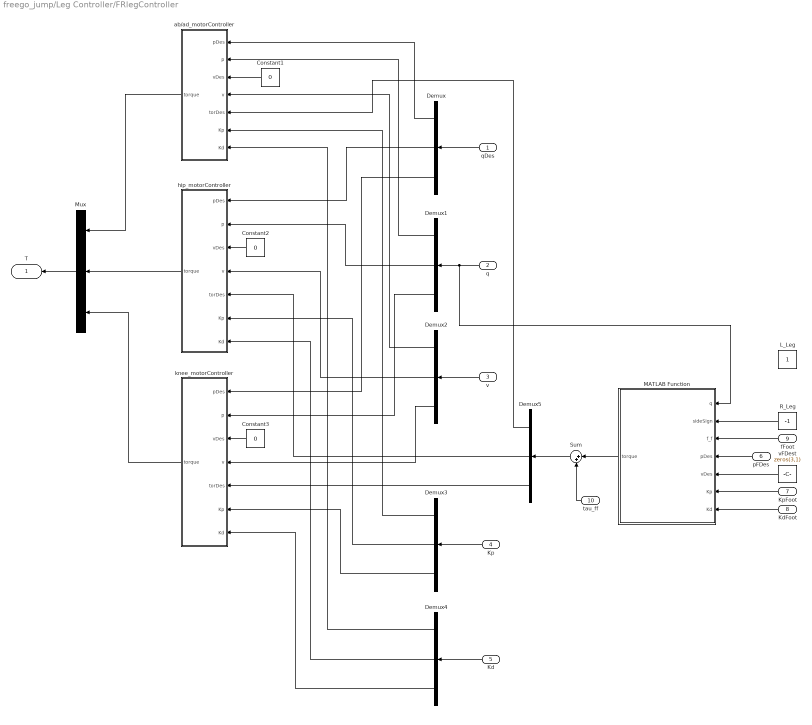
== system freego_jump/Leg Controller/FRlegController ==
  qDes : Inport
  q : Inport  Port=2
  v : Inport  Port=3
  Kp : Inport  Port=4
  Kd : Inport  Port=5
  pFDes : Inport  Port=6
  KpFoot : Inport  Port=7
  KdFoot : Inport  Port=8
  fFoot : Inport  Port=9
  tau_ff : Inport  Port=10
  Constant1 : Constant  Value=0
  Constant2 : Constant  Value=0
  Constant3 : Constant  Value=0
  Demux{,1..5} (6 alike) : Demux  Outputs=3
  L_Leg : Constant
  MATLAB Function : MATLAB Function  TreatAsAtomicUnit=on
  Mux : Mux  Inputs=3
  R_Leg : Constant  Value=-1
  Sum : Sum  Inputs=|++
  ab/ad_motorController : Subsystem
  hip_motorController : Subsystem
  knee_motorController : Subsystem
  vFDest : Constant  Value=zeros(3,1)
  T : Outport
  wires:
  Demux/1 -> ab/ad_motorController/1(pDes)
  Demux1/1 -> ab/ad_motorController/2(p)
  Demux2/1 -> ab/ad_motorController/4(v)
  Demux3/1 -> ab/ad_motorController/6(Kp)
  Demux5/1 -> ab/ad_motorController/5(torDes)
  Constant1/1 -> ab/ad_motorController/3(vDes)
  Demux4/1 -> ab/ad_motorController/7(Kd)
  ab/ad_motorController/1(torque) -> Mux/1
  Constant2/1 -> hip_motorController/3(vDes)
  Demux2/2 -> hip_motorController/4(v)
  Demux/2 -> hip_motorController/1(pDes)
  Demux1/3 -> knee_motorController/2(p)
  Demux5/2 -> hip_motorController/5(torDes)
  Demux3/2 -> hip_motorController/6(Kp)
  Demux5/3 -> knee_motorController/5(torDes)
  Demux/3 -> knee_motorController/1(pDes)
  Constant3/1 -> knee_motorController/3(vDes)
  Demux4/2 -> hip_motorController/7(Kd)
  hip_motorController/1(torque) -> Mux/2
  Demux3/3 -> knee_motorController/6(Kp)
  Demux1/2 -> hip_motorController/2(p)
  knee_motorController/1(torque) -> Mux/3
  Demux4/3 -> knee_motorController/7(Kd)
  qDes/1 -> Demux/1
  q/1 -> MATLAB Function/1(q), Demux1/1
  v/1 -> Demux2/1
  Demux2/3 -> knee_motorController/4(v)
  Kp/1 -> Demux3/1
  Kd/1 -> Demux4/1
  Mux/1 -> T/1
  fFoot/1 -> MATLAB Function/3(f_f)
  KdFoot/1 -> MATLAB Function/7(Kd)
  KpFoot/1 -> MATLAB Function/6(Kp)
  vFDest/1 -> MATLAB Function/5(vDes)
  pFDes/1 -> MATLAB Function/4(pDes)
  MATLAB Function/1(torque) -> Sum/1
  R_Leg/1 -> MATLAB Function/2(sideSign)
  tau_ff/1 -> Sum/2
  Sum/1 -> Demux5/1

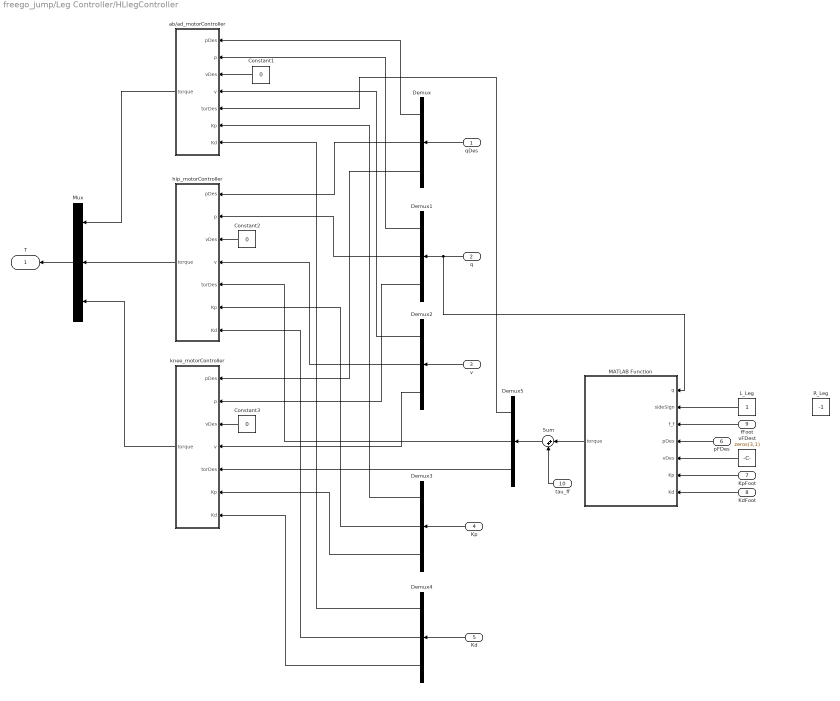
== system freego_jump/Leg Controller/HLlegController ==
  qDes : Inport
  q : Inport  Port=2
  v : Inport  Port=3
  Kp : Inport  Port=4
  Kd : Inport  Port=5
  pFDes : Inport  Port=6
  KpFoot : Inport  Port=7
  KdFoot : Inport  Port=8
  fFoot : Inport  Port=9
  tau_ff : Inport  Port=10
  Constant1 : Constant  Value=0
  Constant2 : Constant  Value=0
  Constant3 : Constant  Value=0
  Demux{,1..5} (6 alike) : Demux  Outputs=3
  L_Leg : Constant
  MATLAB Function : MATLAB Function  TreatAsAtomicUnit=on
  Mux : Mux  Inputs=3
  R_Leg : Constant  Value=-1
  Sum : Sum  Inputs=|++
  ab/ad_motorController : Subsystem
  hip_motorController : Subsystem
  knee_motorController : Subsystem
  vFDest : Constant  Value=zeros(3,1)
  T : Outport
  wires:
  Demux/1 -> ab/ad_motorController/1(pDes)
  Demux1/1 -> ab/ad_motorController/2(p)
  Demux2/1 -> ab/ad_motorController/4(v)
  Demux3/1 -> ab/ad_motorController/6(Kp)
  Demux5/1 -> ab/ad_motorController/5(torDes)
  Constant1/1 -> ab/ad_motorController/3(vDes)
  Demux4/1 -> ab/ad_motorController/7(Kd)
  ab/ad_motorController/1(torque) -> Mux/1
  Constant2/1 -> hip_motorController/3(vDes)
  Demux2/2 -> hip_motorController/4(v)
  Demux/2 -> hip_motorController/1(pDes)
  Demux1/3 -> knee_motorController/2(p)
  Demux5/2 -> hip_motorController/5(torDes)
  Demux3/2 -> hip_motorController/6(Kp)
  Demux5/3 -> knee_motorController/5(torDes)
  Demux/3 -> knee_motorController/1(pDes)
  Constant3/1 -> knee_motorController/3(vDes)
  Demux4/2 -> hip_motorController/7(Kd)
  hip_motorController/1(torque) -> Mux/2
  Demux3/3 -> knee_motorController/6(Kp)
  Demux1/2 -> hip_motorController/2(p)
  knee_motorController/1(torque) -> Mux/3
  Demux4/3 -> knee_motorController/7(Kd)
  qDes/1 -> Demux/1
  q/1 -> MATLAB Function/1(q), Demux1/1
  v/1 -> Demux2/1
  Demux2/3 -> knee_motorController/4(v)
  Kp/1 -> Demux3/1
  Kd/1 -> Demux4/1
  Mux/1 -> T/1
  fFoot/1 -> MATLAB Function/3(f_f)
  KdFoot/1 -> MATLAB Function/7(Kd)
  KpFoot/1 -> MATLAB Function/6(Kp)
  vFDest/1 -> MATLAB Function/5(vDes)
  pFDes/1 -> MATLAB Function/4(pDes)
  L_Leg/1 -> MATLAB Function/2(sideSign)
  tau_ff/1 -> Sum/2
  MATLAB Function/1(torque) -> Sum/1
  Sum/1 -> Demux5/1

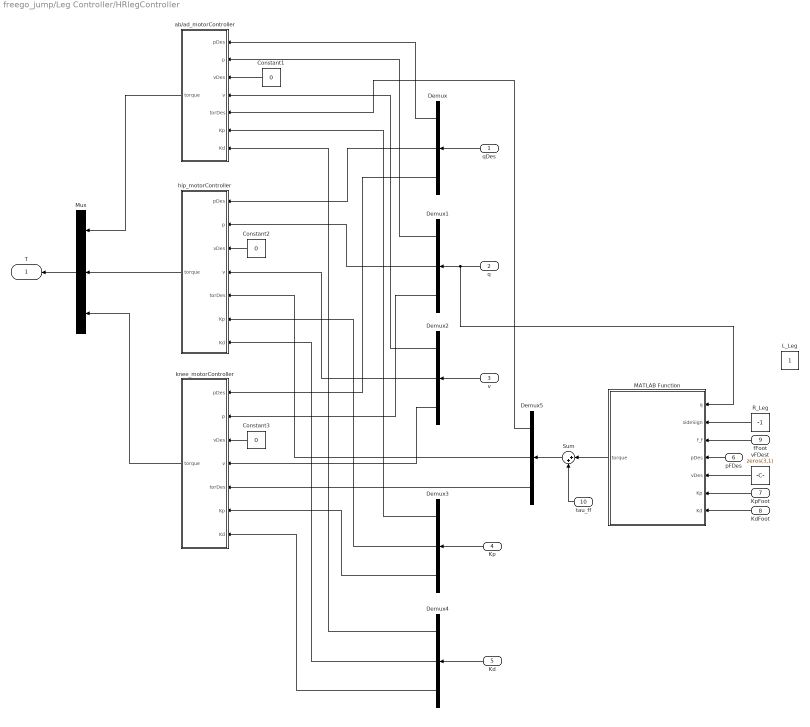
== system freego_jump/Leg Controller/HRlegController ==
  qDes : Inport
  q : Inport  Port=2
  v : Inport  Port=3
  Kp : Inport  Port=4
  Kd : Inport  Port=5
  pFDes : Inport  Port=6
  KpFoot : Inport  Port=7
  KdFoot : Inport  Port=8
  fFoot : Inport  Port=9
  tau_ff : Inport  Port=10
  Constant1 : Constant  Value=0
  Constant2 : Constant  Value=0
  Constant3 : Constant  Value=0
  Demux{,1..5} (6 alike) : Demux  Outputs=3
  L_Leg : Constant
  MATLAB Function : MATLAB Function  TreatAsAtomicUnit=on
  Mux : Mux  Inputs=3
  R_Leg : Constant  Value=-1
  Sum : Sum  Inputs=|++
  ab/ad_motorController : Subsystem
  hip_motorController : Subsystem
  knee_motorController : Subsystem
  vFDest : Constant  Value=zeros(3,1)
  T : Outport
  wires:
  Demux/1 -> ab/ad_motorController/1(pDes)
  Demux1/1 -> ab/ad_motorController/2(p)
  Demux2/1 -> ab/ad_motorController/4(v)
  Demux3/1 -> ab/ad_motorController/6(Kp)
  Demux5/1 -> ab/ad_motorController/5(torDes)
  Constant1/1 -> ab/ad_motorController/3(vDes)
  Demux4/1 -> ab/ad_motorController/7(Kd)
  ab/ad_motorController/1(torque) -> Mux/1
  Constant2/1 -> hip_motorController/3(vDes)
  Demux2/2 -> hip_motorController/4(v)
  Demux/2 -> hip_motorController/1(pDes)
  Demux1/3 -> knee_motorController/2(p)
  Demux5/2 -> hip_motorController/5(torDes)
  Demux3/2 -> hip_motorController/6(Kp)
  Demux5/3 -> knee_motorController/5(torDes)
  Demux/3 -> knee_motorController/1(pDes)
  Constant3/1 -> knee_motorController/3(vDes)
  Demux4/2 -> hip_motorController/7(Kd)
  hip_motorController/1(torque) -> Mux/2
  Demux3/3 -> knee_motorController/6(Kp)
  Demux1/2 -> hip_motorController/2(p)
  knee_motorController/1(torque) -> Mux/3
  Demux4/3 -> knee_motorController/7(Kd)
  qDes/1 -> Demux/1
  q/1 -> MATLAB Function/1(q), Demux1/1
  v/1 -> Demux2/1
  Demux2/3 -> knee_motorController/4(v)
  Kp/1 -> Demux3/1
  Kd/1 -> Demux4/1
  Mux/1 -> T/1
  fFoot/1 -> MATLAB Function/3(f_f)
  KdFoot/1 -> MATLAB Function/7(Kd)
  KpFoot/1 -> MATLAB Function/6(Kp)
  vFDest/1 -> MATLAB Function/5(vDes)
  pFDes/1 -> MATLAB Function/4(pDes)
  R_Leg/1 -> MATLAB Function/2(sideSign)
  tau_ff/1 -> Sum/2
  MATLAB Function/1(torque) -> Sum/1
  Sum/1 -> Demux5/1

== system freego_jump/Subsystem1/LADRC_Pitch ==
  des : Inport
  y : Inport  Port=2
  1/b0 : Gain  Gain=0.5
  Constant2 : Constant  Value=0
  LESO3 : Subsystem
  Sum1 : Sum  Inputs=|+-
  Sum2 : Sum  Inputs=|+-
  Sum3 : Sum  Inputs=+|+
  Sum4 : Sum  Inputs=|+-
  Zero-Pole : ZeroPole  Zeros=[0]  Poles=[-100]  Gain=[100]
  b0 : Gain  Gain=4
  body_atti{,1..3} (4 alike) : Scope  NumInputPorts=2
  d : Gain  Gain=6
  p : Gain  Gain=5
  u : Outport
  wires:
  Sum3/1 -> Sum4/1
  1/b0/1 -> body_atti2/2
  d/1 -> Sum3/2
  y/1 -> Zero-Pole/1, body_atti/2, LESO3/1(y)
  Sum2/1 -> d/1
  LESO3/3(z3) -> 1/b0/1
  p/1 -> Sum3/1
  LESO3/2(z2) -> body_atti2/1
  Sum1/1 -> p/1
  b0/1 -> LESO3/2(b0u)
  LESO3/1(z1) -> body_atti/1, Sum1/2
  Sum4/1 -> body_atti3/2, u/1, b0/1
  des/1 -> Sum1/1, body_atti1/1
  Constant2/1 -> Sum2/1, body_atti1/2
  Zero-Pole/1 -> Sum2/2

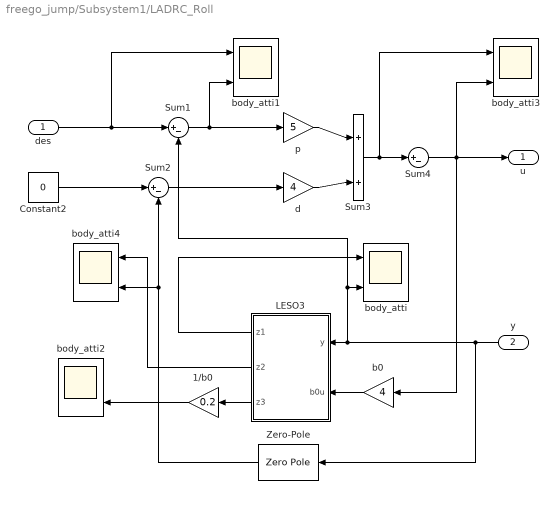
== system freego_jump/Subsystem1/LADRC_Roll ==
  des : Inport
  y : Inport  Port=2
  1/b0 : Gain  Gain=0.2
  Constant2 : Constant  Value=0
  LESO3 : Subsystem
  Sum1 : Sum  Inputs=|+-
  Sum2 : Sum  Inputs=|+-
  Sum3 : Sum  Inputs=+|+
  Sum4 : Sum  Inputs=|+-
  Zero-Pole : ZeroPole  Zeros=[0]  Poles=[-100]  Gain=[100]
  b0 : Gain  Gain=4
  body_atti{,1..4} (5 alike) : Scope  NumInputPorts=2
  d : Gain  Gain=4
  p : Gain  Gain=5
  u : Outport
  wires:
  Sum3/1 -> body_atti3/1, Sum4/1
  1/b0/1 -> body_atti2/2
  d/1 -> Sum3/2
  y/1 -> Zero-Pole/1, Sum1/2, body_atti/2, LESO3/1(y)
  Sum2/1 -> d/1
  LESO3/3(z3) -> 1/b0/1
  p/1 -> Sum3/1
  LESO3/2(z2) -> body_atti4/1
  Sum1/1 -> body_atti1/2, p/1
  b0/1 -> LESO3/2(b0u)
  LESO3/1(z1) -> body_atti/1
  Sum4/1 -> body_atti3/2, u/1, b0/1
  des/1 -> body_atti1/1, Sum1/1
  Constant2/1 -> Sum2/1
  Zero-Pole/1 -> body_atti4/2, Sum2/2

== system freego_jump/Subsystem1/LADRC_Yaw ==
  des : Inport
  y : Inport  Port=2
  1/b0 : Gain  Gain=0.5
  Constant2 : Constant  Value=0
  LESO3 : Subsystem
  Sum1 : Sum  Inputs=|+-
  Sum2 : Sum  Inputs=|+-
  Sum3 : Sum  Inputs=+|+
  Sum4 : Sum  Inputs=|+-
  Zero-Pole : ZeroPole  Zeros=[0]  Poles=[-100]  Gain=[100]
  b0 : Gain  Gain=2
  body_atti : Scope  NumInputPorts=2
  body_atti1 : Scope  NumInputPorts=2
  body_atti2 : Scope  NumInputPorts=2
  d : Gain  Gain=4
  p : Gain  Gain=3
  u : Outport
  wires:
  Sum3/1 -> Sum4/1
  1/b0/1 -> body_atti2/2
  d/1 -> Sum3/2
  y/1 -> Zero-Pole/1, Sum1/2, body_atti/2, LESO3/1(y)
  Sum2/1 -> d/1
  LESO3/3(z3) -> 1/b0/1
  p/1 -> Sum3/1
  LESO3/2(z2) -> body_atti2/1
  Sum1/1 -> p/1
  b0/1 -> LESO3/2(b0u)
  LESO3/1(z1) -> body_atti/1
  Sum4/1 -> u/1, b0/1
  des/1 -> Sum1/1, body_atti1/1
  Constant2/1 -> Sum2/1, body_atti1/2
  Zero-Pole/1 -> Sum2/2

== system freego_jump/Leg Controller/FLlegController/ab//ad_motorController ==
  pDes : Inport
  p : Inport  Port=2
  vDes : Inport  Port=3
  v : Inport  Port=4
  torDes : Inport  Port=5
  Kp : Inport  Port=6
  Kd : Inport  Port=7
  Product : Product
  Product1 : Product
  Sum1 : Sum  Inputs=|+-
  Sum2 : Sum  Inputs=|+-
  Sum3 : Sum  Inputs=+++
  torque : Outport
  wires:
  Sum1/1 -> Product1/1
  Product/1 -> Sum3/1
  vDes/1 -> Sum1/1
  v/1 -> Sum1/2
  p/1 -> Sum2/2
  Sum3/1 -> torque/1
  pDes/1 -> Sum2/1
  Sum2/1 -> Product/2
  Product1/1 -> Sum3/2
  torDes/1 -> Sum3/3
  Kp/1 -> Product/1
  Kd/1 -> Product1/2

== system freego_jump/Leg Controller/FLlegController/hip_motorController ==
  pDes : Inport
  p : Inport  Port=2
  vDes : Inport  Port=3
  v : Inport  Port=4
  torDes : Inport  Port=5
  Kp : Inport  Port=6
  Kd : Inport  Port=7
  Product : Product
  Product1 : Product
  Sum1 : Sum  Inputs=|+-
  Sum2 : Sum  Inputs=|+-
  Sum3 : Sum  Inputs=+++
  torque : Outport
  wires:
  Sum1/1 -> Product1/1
  Product/1 -> Sum3/1
  vDes/1 -> Sum1/1
  v/1 -> Sum1/2
  p/1 -> Sum2/2
  Sum3/1 -> torque/1
  pDes/1 -> Sum2/1
  Sum2/1 -> Product/2
  Product1/1 -> Sum3/2
  torDes/1 -> Sum3/3
  Kp/1 -> Product/1
  Kd/1 -> Product1/2

== system freego_jump/Leg Controller/FLlegController/knee_motorController ==
  pDes : Inport
  p : Inport  Port=2
  vDes : Inport  Port=3
  v : Inport  Port=4
  torDes : Inport  Port=5
  Kp : Inport  Port=6
  Kd : Inport  Port=7
  Product : Product
  Product1 : Product
  Sum1 : Sum  Inputs=|+-
  Sum2 : Sum  Inputs=|+-
  Sum3 : Sum  Inputs=+++
  torque : Outport
  wires:
  Sum1/1 -> Product1/1
  Product/1 -> Sum3/1
  vDes/1 -> Sum1/1
  v/1 -> Sum1/2
  p/1 -> Sum2/2
  Sum3/1 -> torque/1
  pDes/1 -> Sum2/1
  Sum2/1 -> Product/2
  Product1/1 -> Sum3/2
  torDes/1 -> Sum3/3
  Kp/1 -> Product/1
  Kd/1 -> Product1/2

== system freego_jump/Leg Controller/FRlegController/ab//ad_motorController ==
  pDes : Inport
  p : Inport  Port=2
  vDes : Inport  Port=3
  v : Inport  Port=4
  torDes : Inport  Port=5
  Kp : Inport  Port=6
  Kd : Inport  Port=7
  Product : Product
  Product1 : Product
  Sum1 : Sum  Inputs=|+-
  Sum2 : Sum  Inputs=|+-
  Sum3 : Sum  Inputs=+++
  torque : Outport
  wires:
  Sum1/1 -> Product1/1
  Product/1 -> Sum3/1
  vDes/1 -> Sum1/1
  v/1 -> Sum1/2
  p/1 -> Sum2/2
  Sum3/1 -> torque/1
  pDes/1 -> Sum2/1
  Sum2/1 -> Product/2
  Product1/1 -> Sum3/2
  torDes/1 -> Sum3/3
  Kp/1 -> Product/1
  Kd/1 -> Product1/2

== system freego_jump/Leg Controller/FRlegController/hip_motorController ==
  pDes : Inport
  p : Inport  Port=2
  vDes : Inport  Port=3
  v : Inport  Port=4
  torDes : Inport  Port=5
  Kp : Inport  Port=6
  Kd : Inport  Port=7
  Product : Product
  Product1 : Product
  Sum1 : Sum  Inputs=|+-
  Sum2 : Sum  Inputs=|+-
  Sum3 : Sum  Inputs=+++
  torque : Outport
  wires:
  Sum1/1 -> Product1/1
  Product/1 -> Sum3/1
  vDes/1 -> Sum1/1
  v/1 -> Sum1/2
  p/1 -> Sum2/2
  Sum3/1 -> torque/1
  pDes/1 -> Sum2/1
  Sum2/1 -> Product/2
  Product1/1 -> Sum3/2
  torDes/1 -> Sum3/3
  Kp/1 -> Product/1
  Kd/1 -> Product1/2

== system freego_jump/Leg Controller/FRlegController/knee_motorController ==
  pDes : Inport
  p : Inport  Port=2
  vDes : Inport  Port=3
  v : Inport  Port=4
  torDes : Inport  Port=5
  Kp : Inport  Port=6
  Kd : Inport  Port=7
  Product : Product
  Product1 : Product
  Sum1 : Sum  Inputs=|+-
  Sum2 : Sum  Inputs=|+-
  Sum3 : Sum  Inputs=+++
  torque : Outport
  wires:
  Sum1/1 -> Product1/1
  Product/1 -> Sum3/1
  vDes/1 -> Sum1/1
  v/1 -> Sum1/2
  p/1 -> Sum2/2
  Sum3/1 -> torque/1
  pDes/1 -> Sum2/1
  Sum2/1 -> Product/2
  Product1/1 -> Sum3/2
  torDes/1 -> Sum3/3
  Kp/1 -> Product/1
  Kd/1 -> Product1/2

== system freego_jump/Leg Controller/HLlegController/ab//ad_motorController ==
  pDes : Inport
  p : Inport  Port=2
  vDes : Inport  Port=3
  v : Inport  Port=4
  torDes : Inport  Port=5
  Kp : Inport  Port=6
  Kd : Inport  Port=7
  Product : Product
  Product1 : Product
  Sum1 : Sum  Inputs=|+-
  Sum2 : Sum  Inputs=|+-
  Sum3 : Sum  Inputs=+++
  torque : Outport
  wires:
  Sum1/1 -> Product1/1
  Product/1 -> Sum3/1
  vDes/1 -> Sum1/1
  v/1 -> Sum1/2
  p/1 -> Sum2/2
  Sum3/1 -> torque/1
  pDes/1 -> Sum2/1
  Sum2/1 -> Product/2
  Product1/1 -> Sum3/2
  torDes/1 -> Sum3/3
  Kp/1 -> Product/1
  Kd/1 -> Product1/2

== system freego_jump/Leg Controller/HLlegController/hip_motorController ==
  pDes : Inport
  p : Inport  Port=2
  vDes : Inport  Port=3
  v : Inport  Port=4
  torDes : Inport  Port=5
  Kp : Inport  Port=6
  Kd : Inport  Port=7
  Product : Product
  Product1 : Product
  Sum1 : Sum  Inputs=|+-
  Sum2 : Sum  Inputs=|+-
  Sum3 : Sum  Inputs=+++
  torque : Outport
  wires:
  Sum1/1 -> Product1/1
  Product/1 -> Sum3/1
  vDes/1 -> Sum1/1
  v/1 -> Sum1/2
  p/1 -> Sum2/2
  Sum3/1 -> torque/1
  pDes/1 -> Sum2/1
  Sum2/1 -> Product/2
  Product1/1 -> Sum3/2
  torDes/1 -> Sum3/3
  Kp/1 -> Product/1
  Kd/1 -> Product1/2

== system freego_jump/Leg Controller/HLlegController/knee_motorController ==
  pDes : Inport
  p : Inport  Port=2
  vDes : Inport  Port=3
  v : Inport  Port=4
  torDes : Inport  Port=5
  Kp : Inport  Port=6
  Kd : Inport  Port=7
  Product : Product
  Product1 : Product
  Sum1 : Sum  Inputs=|+-
  Sum2 : Sum  Inputs=|+-
  Sum3 : Sum  Inputs=+++
  torque : Outport
  wires:
  Sum1/1 -> Product1/1
  Product/1 -> Sum3/1
  vDes/1 -> Sum1/1
  v/1 -> Sum1/2
  p/1 -> Sum2/2
  Sum3/1 -> torque/1
  pDes/1 -> Sum2/1
  Sum2/1 -> Product/2
  Product1/1 -> Sum3/2
  torDes/1 -> Sum3/3
  Kp/1 -> Product/1
  Kd/1 -> Product1/2

== system freego_jump/Leg Controller/HRlegController/ab//ad_motorController ==
  pDes : Inport
  p : Inport  Port=2
  vDes : Inport  Port=3
  v : Inport  Port=4
  torDes : Inport  Port=5
  Kp : Inport  Port=6
  Kd : Inport  Port=7
  Product : Product
  Product1 : Product
  Sum1 : Sum  Inputs=|+-
  Sum2 : Sum  Inputs=|+-
  Sum3 : Sum  Inputs=+++
  torque : Outport
  wires:
  Sum1/1 -> Product1/1
  Product/1 -> Sum3/1
  vDes/1 -> Sum1/1
  v/1 -> Sum1/2
  p/1 -> Sum2/2
  Sum3/1 -> torque/1
  pDes/1 -> Sum2/1
  Sum2/1 -> Product/2
  Product1/1 -> Sum3/2
  torDes/1 -> Sum3/3
  Kp/1 -> Product/1
  Kd/1 -> Product1/2

== system freego_jump/Leg Controller/HRlegController/hip_motorController ==
  pDes : Inport
  p : Inport  Port=2
  vDes : Inport  Port=3
  v : Inport  Port=4
  torDes : Inport  Port=5
  Kp : Inport  Port=6
  Kd : Inport  Port=7
  Product : Product
  Product1 : Product
  Sum1 : Sum  Inputs=|+-
  Sum2 : Sum  Inputs=|+-
  Sum3 : Sum  Inputs=+++
  torque : Outport
  wires:
  Sum1/1 -> Product1/1
  Product/1 -> Sum3/1
  vDes/1 -> Sum1/1
  v/1 -> Sum1/2
  p/1 -> Sum2/2
  Sum3/1 -> torque/1
  pDes/1 -> Sum2/1
  Sum2/1 -> Product/2
  Product1/1 -> Sum3/2
  torDes/1 -> Sum3/3
  Kp/1 -> Product/1
  Kd/1 -> Product1/2

== system freego_jump/Leg Controller/HRlegController/knee_motorController ==
  pDes : Inport
  p : Inport  Port=2
  vDes : Inport  Port=3
  v : Inport  Port=4
  torDes : Inport  Port=5
  Kp : Inport  Port=6
  Kd : Inport  Port=7
  Product : Product
  Product1 : Product
  Sum1 : Sum  Inputs=|+-
  Sum2 : Sum  Inputs=|+-
  Sum3 : Sum  Inputs=+++
  torque : Outport
  wires:
  Sum1/1 -> Product1/1
  Product/1 -> Sum3/1
  vDes/1 -> Sum1/1
  v/1 -> Sum1/2
  p/1 -> Sum2/2
  Sum3/1 -> torque/1
  pDes/1 -> Sum2/1
  Sum2/1 -> Product/2
  Product1/1 -> Sum3/2
  torDes/1 -> Sum3/3
  Kp/1 -> Product/1
  Kd/1 -> Product1/2

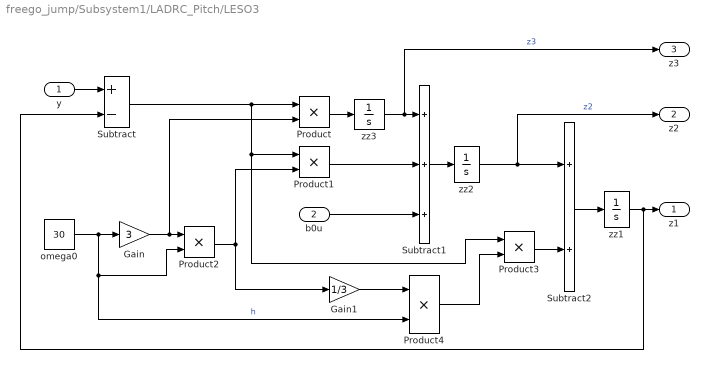
== system freego_jump/Subsystem1/LADRC_Pitch/LESO3 ==
  y : Inport
  b0u : Inport  Port=2
  Gain : Gain  Gain=3
  Gain1 : Gain  Gain=1/3
  Product{,1..4} (5 alike) : Product
  Subtract : Sum  Inputs=+-
  Subtract1 : Sum  Inputs=+++
  Subtract2 : Sum
  omega0 : Constant  Value=30
  zz1 : Integrator
  zz2 : Integrator
  zz3 : Integrator
  z1 : Outport
  z2 : Outport  Port=2
  z3 : Outport  Port=3
  wires:
  y/1 -> Subtract/1
  Subtract/1 -> Product/1, Product3/1, Product1/1
  omega0/1 -> Gain/1, Product4/2, Product2/2  "h"
  Gain/1 -> Product/2, Product2/1
  Product/1 -> zz3/1
  zz3/1 -> z3/1, Subtract1/1  "z3"
  b0u/1 -> Subtract1/3
  Product1/1 -> Subtract1/2
  Product2/1 -> Gain1/1, Product1/2
  Subtract1/1 -> zz2/1
  zz2/1 -> Subtract2/1, z2/1  "z2"
  zz1/1 -> Subtract/2, z1/1
  Product3/1 -> Subtract2/2
  Product4/1 -> Product3/2
  Subtract2/1 -> zz1/1
  Gain1/1 -> Product4/1

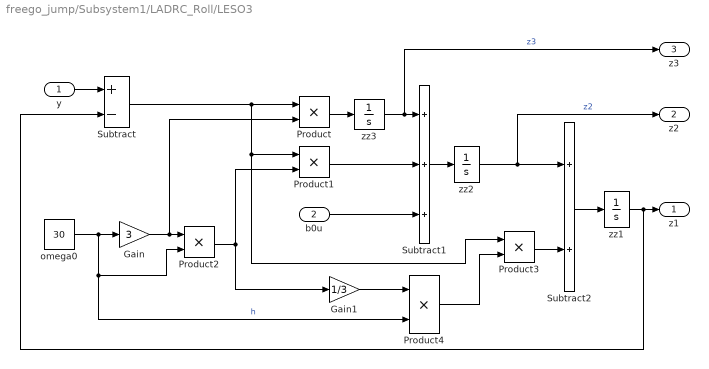
== system freego_jump/Subsystem1/LADRC_Roll/LESO3 ==
  y : Inport
  b0u : Inport  Port=2
  Gain : Gain  Gain=3
  Gain1 : Gain  Gain=1/3
  Product{,1..4} (5 alike) : Product
  Subtract : Sum  Inputs=+-
  Subtract1 : Sum  Inputs=+++
  Subtract2 : Sum
  omega0 : Constant  Value=30
  zz1 : Integrator
  zz2 : Integrator
  zz3 : Integrator
  z1 : Outport
  z2 : Outport  Port=2
  z3 : Outport  Port=3
  wires:
  y/1 -> Subtract/1
  Subtract/1 -> Product/1, Product3/1, Product1/1
  omega0/1 -> Gain/1, Product4/2, Product2/2  "h"
  Gain/1 -> Product/2, Product2/1
  Product/1 -> zz3/1
  zz3/1 -> z3/1, Subtract1/1  "z3"
  b0u/1 -> Subtract1/3
  Product1/1 -> Subtract1/2
  Product2/1 -> Gain1/1, Product1/2
  Subtract1/1 -> zz2/1
  zz2/1 -> Subtract2/1, z2/1  "z2"
  zz1/1 -> Subtract/2, z1/1
  Product3/1 -> Subtract2/2
  Product4/1 -> Product3/2
  Subtract2/1 -> zz1/1
  Gain1/1 -> Product4/1

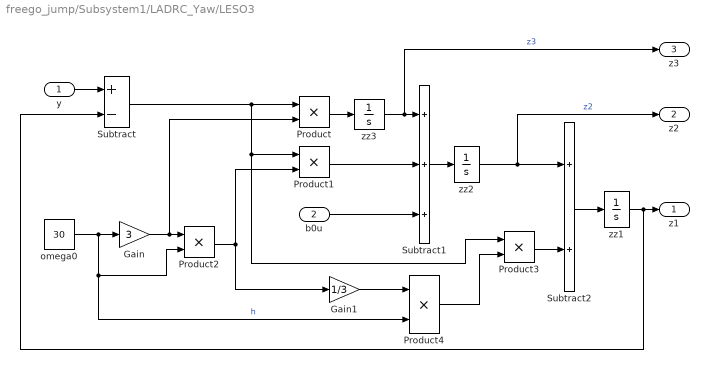
== system freego_jump/Subsystem1/LADRC_Yaw/LESO3 ==
  y : Inport
  b0u : Inport  Port=2
  Gain : Gain  Gain=3
  Gain1 : Gain  Gain=1/3
  Product{,1..4} (5 alike) : Product
  Subtract : Sum  Inputs=+-
  Subtract1 : Sum  Inputs=+++
  Subtract2 : Sum
  omega0 : Constant  Value=30
  zz1 : Integrator
  zz2 : Integrator
  zz3 : Integrator
  z1 : Outport
  z2 : Outport  Port=2
  z3 : Outport  Port=3
  wires:
  y/1 -> Subtract/1
  Subtract/1 -> Product/1, Product3/1, Product1/1
  omega0/1 -> Gain/1, Product4/2, Product2/2  "h"
  Gain/1 -> Product/2, Product2/1
  Product/1 -> zz3/1
  zz3/1 -> z3/1, Subtract1/1  "z3"
  b0u/1 -> Subtract1/3
  Product1/1 -> Subtract1/2
  Product2/1 -> Gain1/1, Product1/2
  Subtract1/1 -> zz2/1
  zz2/1 -> Subtract2/1, z2/1  "z2"
  zz1/1 -> Subtract/2, z1/1
  Product3/1 -> Subtract2/2
  Product4/1 -> Product3/2
  Subtract2/1 -> zz1/1
  Gain1/1 -> Product4/1

== matlab function freego_jump/TD/MATLAB Function1 ==
  data: x1 input; fh output; x2 input; r input; h input
function  fh = fhan(x1, x2, r, h)
     d = r*h;
     d0 = h*d;
     y = x1 + h*x2;
     a0 = sqrt(d*d +8*r*abs(y));
     
     if abs(y)>d0
         a = x2 + (a0 - d)*sign(y)/2;
     else 
         a = x2 + y/h;
     end
     
     if abs(a)>d
         fh = -r*sign(a);
     else
         fh = -r*a/d;
     end
end

== matlab function freego_jump/LADRC/TD3 /MATLAB Function1 ==
  data: x1 input; x2 input; f output; u input; r input; d input
function f = fst2(x1, x2, u, r, d)
v=x1-u+abs(x2)*x2/(2*r);
if v>=d
    f=sign(v);
else f=v/d;
end
